simulink subsystem "Sub_Plant_And_Environments"  (R2020a)
settings: Solver=VariableStepAuto  StartTime=0.0  StopTime=10.0  RelTol=1e-3
values from neighbouring files (symbols this model uses):
  a_rad = deg2rad(a)    [plant_init.m]
  AF = [0.12, 0.22, 0.292]    [plant_init.m]
  l1 = [(D14(3)-RB(3)+PZ(1)*dz),     (D14(3)-RB(3)+PZ(1)*dz),     -hypot( D14(1)-RB(1), D14(2)-RB(2))]    [plant_init.m]
  l2 = [-(D14(3)-RB(3)+PZ(2)*dz),      (D14(3)-RB(3)+PZ(2)*dz),      -hypot( D14(1)+RB(1), D14(2)-RB(2))]    [plant_init.m]
  l3 = [(D14(3)-RB(3)+PZ(3)*dz),      (D14(3)-RB(3)+PZ(3)*dz),      hypot(D14(1)+RB(1), D14(2)+RB(2))]    [plant_init.m]
  l4 = [-(D14(3)-RB(3)+PZ(4)*dz),      (D14(3)-RB(3)+PZ(4)*dz),      hypot(D14(1)-RB(1), D14(2)+RB(2))]    [plant_init.m]
  l5 = [(D58(2)-RB(2)+PZ(1)*dz),      -(D58(1)-RB(1)+PZ(1)*dz), 0]    [plant_init.m]
  l6 = [-(D58(2)-RB(2)+PZ(2)*dz),       -(D58(1)+RB(1)+PZ(2)*dz), 0]    [plant_init.m]
  l7 = [-(D58(2)+RB(2)+PZ(3)*dz),     (D58(1)+RB(1)+PZ(3)*dz), 0]    [plant_init.m]
  l8 = [(D58(2)+RB(2)+PZ(4)*dz),      (D58(1)-RB(1)+PZ(2)*dz), 0]    [plant_init.m]
  mass = 33.95    [plant_init.m]
  N = T200Spec16V{:,6}    [InitController.m]    (also in plant_init.m)
  PWM = T200Spec16V{:,1}    [InitController.m]    (also in plant_init.m)
  RB = [ 0.001,      -0.003,       0.027]    [plant_init.m]
  RG = [ 0.001,      -0.003,       0.027]    [plant_init.m]
  rho = 998    [plant_init.m]
  volume = 0.027    [plant_init.m]
libraries: sharedtransform x11, vrlib x9, shared6dof x1, aerolibasang x1
(part 1 of 2)
settings Model: Creator=Lamarre  LastModifiedBy=Lamarre

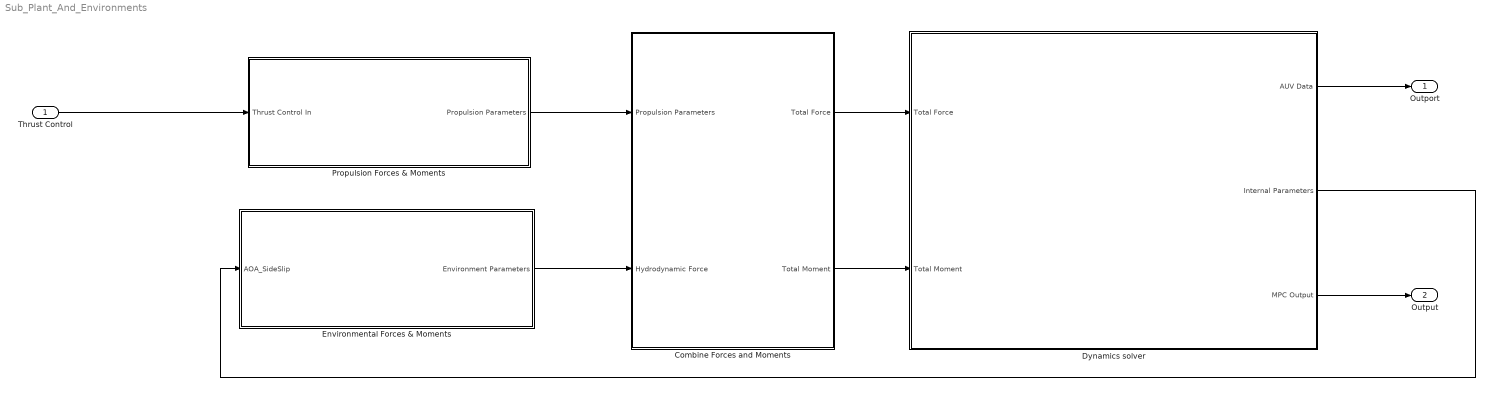
== system Sub_Plant_And_Environments ==
  Thrust Control : Inport
  Combine Forces and Moments : Subsystem
  Dynamics solver : Subsystem
  Environmental Forces & Moments : Subsystem
  Propulsion Forces & Moments : Subsystem
  Outport : Outport  VectorParamsAs1DForOutWhenUnconnected=off
  Output : Outport  Port=2
  wires:
  Dynamics solver/1(AUV Data) -> Outport/1
  Environmental Forces & Moments/1(Environment Parameters) -> Combine Forces and Moments/2(Hydrodynamic Force)
  Dynamics solver/2(Internal Parameters) -> Environmental Forces & Moments/1(AOA_SideSlip)
  Combine Forces and Moments/1(Total Force) -> Dynamics solver/1(Total Force)
  Thrust Control/1 -> Propulsion Forces & Moments/1(Thrust Control In)
  Propulsion Forces & Moments/1(Propulsion Parameters) -> Combine Forces and Moments/1(Propulsion Parameters)
  Dynamics solver/3(MPC Output) -> Output/1
  Combine Forces and Moments/2(Total Moment) -> Dynamics solver/2(Total Moment)

== system Sub_Plant_And_Environments/Combine Forces and Moments ==
  Propulsion Parameters : Inport
  Hydrodynamic Force : Inport  Port=2
  Bus Selector : BusSelector  OutputSignals=PropForce,PropMoment
  Bus Selector1 : BusSelector  OutputSignals=LDForce,HSForce,HS Moment
  Saturation : Saturate  UpperLimit=600  LowerLimit=-600
  Saturation1 : Saturate  UpperLimit=600  LowerLimit=-600
  Sum : Sum  Inputs=+++
  Sum1 : Sum  Inputs=|++
  Total Force : Outport  VectorParamsAs1DForOutWhenUnconnected=off
  Total Moment : Outport  Port=2  VectorParamsAs1DForOutWhenUnconnected=off
  wires:
  Bus Selector1/3 -> Sum1/2  "<HS Moment>"
  Bus Selector/2 -> Sum1/1  "<PropMoment>"
  Sum/1 -> Saturation/1
  Sum1/1 -> Total Moment/1
  Saturation1/1 -> Sum/2
  Saturation/1 -> Total Force/1
  Propulsion Parameters/1 -> Bus Selector/1
  Hydrodynamic Force/1 -> Bus Selector1/1
  Bus Selector/1 -> Sum/1  "<PropForce>"
  Bus Selector1/1 -> Saturation1/1  "<LDForce>"
  Bus Selector1/2 -> Sum/3  "<HSForce>"

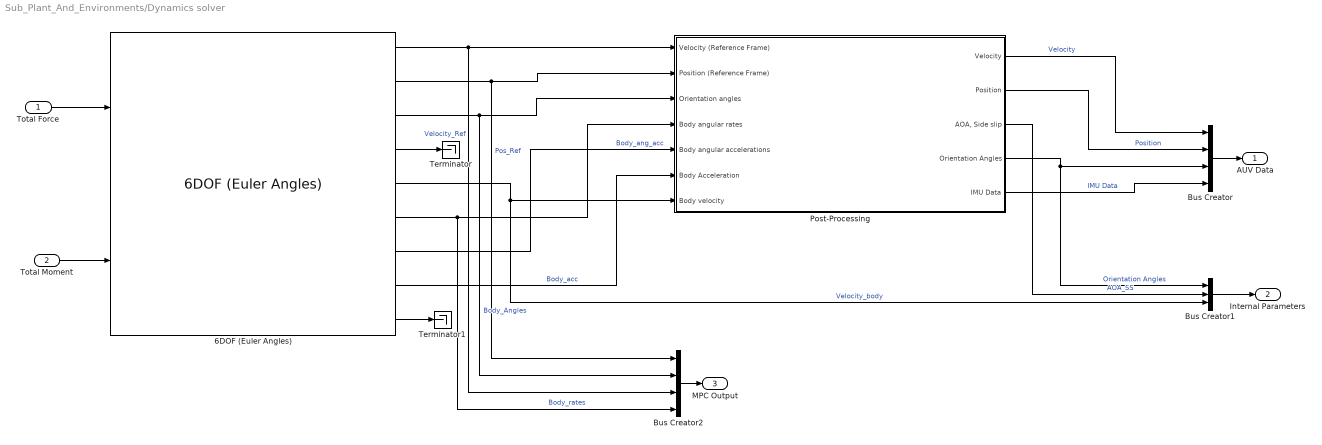
== system Sub_Plant_And_Environments/Dynamics solver ==
  Total Force : Inport
  Total Moment : Inport  Port=2
  6DOF (Euler Angles) : shared6dof/6DOF (Euler Angles)  units=Metric (MKS)  mtype=Fixed  rep=Euler Angles  xme_0=IP  Vm_0=IV  eul_0=IE  pm_0=IB  mass_0=mass  mass_e=0.5  mass_f=2.0  inertia=I  inertia_e=eye(3)  inertia_f=2*eye(3)  k_quat=1.0  vre_flag=on  abi_flag=on  aMode=0  xme_statename=''  Vm_statename=''  eul_statename=''  quat_statename=''  pm_statename=''  mass_statename=''
      settings: SourceProductBaseCode=AE,PW,MT,VE,VP
  Bus Creator : BusCreator  Inputs=4
  Bus Creator1 : BusCreator  Inputs=3
  Bus Creator2 : BusCreator  Inputs=4
  Post-Processing : Subsystem
  Terminator : Terminator
  Terminator1 : Terminator
  AUV Data : Outport  VectorParamsAs1DForOutWhenUnconnected=off
  Internal Parameters : Outport  Port=2  VectorParamsAs1DForOutWhenUnconnected=off
  MPC Output : Outport  Port=3
  wires:
  6DOF (Euler Angles)/6 -> Bus Creator2/4, Post-Processing/4(Body angular rates)  "Body_rates"
  Post-Processing/3("AOA, Side slip") -> Bus Creator1/2  "AOA_SS"
  6DOF (Euler Angles)/8 -> Post-Processing/6(Body Acceleration)  "Body_acc"
  Post-Processing/2(" Position") -> Bus Creator/2  "Position"
  6DOF (Euler Angles)/7 -> Post-Processing/5(Body angular accelerations)  "Body_ang_acc"
  6DOF (Euler Angles)/2 -> Bus Creator2/1, Post-Processing/2(Position (Reference Frame))  "Pos_Ref"
  6DOF (Euler Angles)/3 -> Bus Creator2/2, Post-Processing/3(Orientation angles)  "Body_Angles"
  Post-Processing/1(Velocity) -> Bus Creator/1  "Velocity"
  6DOF (Euler Angles)/1 -> Post-Processing/1(Velocity (Reference Frame)), Bus Creator2/3  "Velocity_Ref"
  6DOF (Euler Angles)/5 -> Bus Creator1/3, Post-Processing/7(Body velocity)  "Velocity_body"
  Post-Processing/4(Orientation Angles) -> Bus Creator1/1, Bus Creator/3  "Orientation Angles"
  Total Force/1 -> 6DOF (Euler Angles)/1
  Total Moment/1 -> 6DOF (Euler Angles)/2
  Bus Creator/1 -> AUV Data/1
  Bus Creator1/1 -> Internal Parameters/1
  6DOF (Euler Angles)/4 -> Terminator/1
  6DOF (Euler Angles)/9 -> Terminator1/1
  Post-Processing/5(IMU Data) -> Bus Creator/4  "IMU Data"
  Bus Creator2/1 -> MPC Output/1

== system Sub_Plant_And_Environments/Environmental Forces & Moments ==
  AOA_SideSlip : Inport
  Bus Creator : BusCreator  Inputs=3
  Bus Selector : BusSelector  OutputSignals=Velocity_body,AOA_SS,Orientation Angles
  Hydrodynamic Forces : Subsystem  Variant=on
  Hydrostatic Forces : Subsystem
  Environment Parameters : Outport  VectorParamsAs1DForOutWhenUnconnected=off
  wires:
  Hydrodynamic Forces/1("Force due to Lift, Drag") -> Bus Creator/1  "LDForce"
  Hydrostatic Forces/1(Hydrostatic Force) -> Bus Creator/2  "HSForce"
  Hydrostatic Forces/2(Hydrostatic Moment) -> Bus Creator/3  "HS Moment"
  Bus Creator/1 -> Environment Parameters/1
  AOA_SideSlip/1 -> Bus Selector/1
  Bus Selector/1 -> Hydrodynamic Forces/1("Submarine Velocity (Body Axis) ")  "<Velocity_body>"
  Bus Selector/2 -> Hydrodynamic Forces/2("AOA, Side Slip")  "<AOA_SS>"
  Bus Selector/3 -> Hydrostatic Forces/1(In1)  "<Orientation Angles>"

== system Sub_Plant_And_Environments/Propulsion Forces & Moments ==
  Thrust Control In : Inport
  Bus Creator : BusCreator  Inputs=2
  Force and moments due to Thrust : Subsystem
  Input commands to Thrust : Subsystem
  Propulsion Parameters : Outport  VectorParamsAs1DForOutWhenUnconnected=off
  wires:
  Input commands to Thrust/1(Thrust values) -> Force and moments due to Thrust/1(Thrust Inputs)
  Thrust Control In/1 -> Input commands to Thrust/1(Thrust Control Inputs)
  Force and moments due to Thrust/1(Propulsion Force) -> Bus Creator/1  "PropForce"
  Force and moments due to Thrust/2(Propulsion Moment) -> Bus Creator/2  "PropMoment"
  Bus Creator/1 -> Propulsion Parameters/1

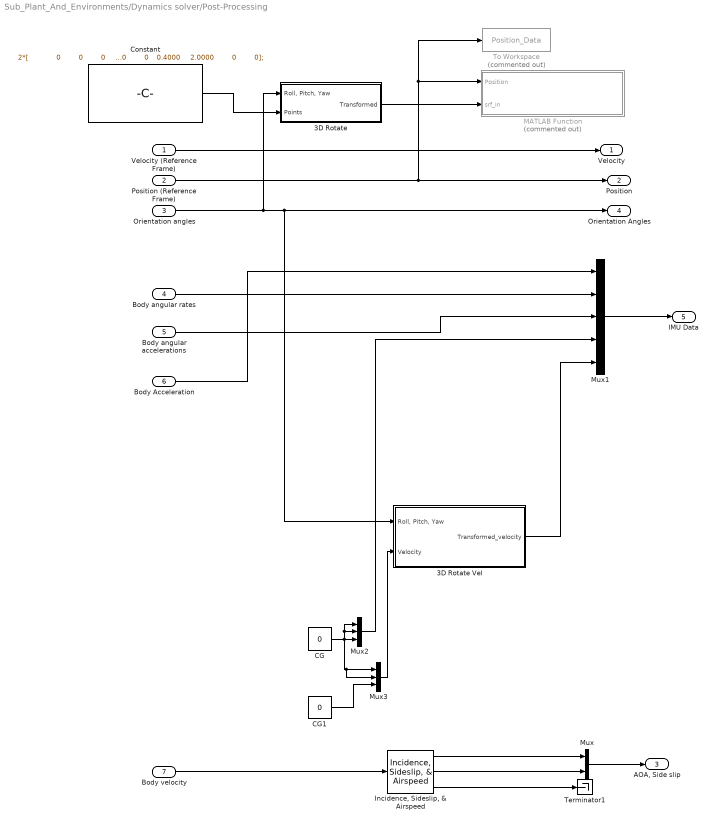
== system Sub_Plant_And_Environments/Dynamics solver/Post-Processing ==
  Velocity (Reference Frame) : Inport
  Position (Reference Frame) : Inport  Port=2
  Orientation angles : Inport  Port=3
  Body angular rates : Inport  Port=4
  Body angular accelerations : Inport  Port=5
  Body Acceleration : Inport  Port=6
  Body velocity : Inport  Port=7
  "3D Rotate " : Subsystem
  3D Rotate Vel : Subsystem
  CG : Constant  Value=0
  CG1 : Constant  Value=0
  Constant : Constant  Value=|
      | 2*[              0         0         0
      |     2.0000         0         0
      |     2.0000    0.4000         0
      |          0    0.4000         0
      |          0         0         0
      |          0         0    0.4000
      |     2.0000         0    0.4000
      |     2.0000    0.4000    0.4000
      |          0    0.4000    0.4000
      |          0         0    0.4000
      |          0    0.4000    0.4000
      |          0    0.4000         0
      |     2.0000    0.4000         0
      |     2.0000    0.4000    0.4000
      |     2.0000         0    0.4000
      |     2.0000         0         0];
  "Incidence, Sideslip, & Airspeed" : aerolibasang/Incidence, Sideslip, & Airspeed
  MATLAB Function : MATLAB Function  Commented=on  TreatAsAtomicUnit=on  SystemSampleTime=0.05
  Mux : Mux  Inputs=2
  Mux1 : Mux  Inputs=5
  Mux2 : Mux  Inputs=3
  Mux3 : Mux  Inputs=3
  Terminator1 : Terminator
  To Workspace : ToWorkspace  Commented=on  VariableName=Position_Data  SampleTime=-1
  Velocity : Outport  VectorParamsAs1DForOutWhenUnconnected=off
  " Position" : Outport  Port=2  VectorParamsAs1DForOutWhenUnconnected=off
  "AOA, Side slip" : Outport  Port=3  VectorParamsAs1DForOutWhenUnconnected=off
  Orientation Angles : Outport  Port=4  VectorParamsAs1DForOutWhenUnconnected=off
  IMU Data : Outport  Port=5  VectorParamsAs1DForOutWhenUnconnected=off
  wires:
  Body angular accelerations/1 -> Mux1/3
  "Incidence, Sideslip, & Airspeed"/2 -> Mux/2
  Body velocity/1 -> "Incidence, Sideslip, & Airspeed"/1
  "Incidence, Sideslip, & Airspeed"/1 -> Mux/1
  Body angular rates/1 -> Mux1/2
  CG/1 -> Mux3/2, Mux3/1, Mux2/3, Mux2/2, Mux2/1
  3D Rotate Vel/1("Transformed_velocity ") -> Mux1/5
  Mux2/1 -> Mux1/4
  Position (Reference Frame)/1 -> To Workspace/1, MATLAB Function/1(Position), " Position"/1
  Mux/1 -> "AOA, Side slip"/1
  CG1/1 -> Mux3/3
  Mux3/1 -> 3D Rotate Vel/2(Velocity)
  Body Acceleration/1 -> Mux1/1
  Velocity (Reference Frame)/1 -> Velocity/1
  Orientation angles/1 -> 3D Rotate Vel/1("Roll, Pitch, Yaw"), Orientation Angles/1, "3D Rotate "/1("Roll, Pitch, Yaw")
  Mux1/1 -> IMU Data/1
  Constant/1 -> "3D Rotate "/2(Points)
  "3D Rotate "/1("Transformed ") -> MATLAB Function/2(srf_in)
  "Incidence, Sideslip, & Airspeed"/3 -> Terminator1/1

== system Sub_Plant_And_Environments/Environmental Forces & Moments/Hydrodynamic Forces ==
  "Submarine Velocity (Body Axis) " : Inport
  "AOA, Side Slip" : Inport  Port=2
  Hydrodynamic Forces - Accurate : Subsystem  VariantControl=c==1
  Hydrodynamic Forces - Basic : Subsystem  VariantControl=c==0
  "Force due to Lift, Drag" : Outport  VectorParamsAs1DForOutWhenUnconnected=off

== system Sub_Plant_And_Environments/Environmental Forces & Moments/Hydrostatic Forces ==
  In1 : Inport
  Constant : Constant
  Environment Model : Subsystem  mask{ro=rho, V=volume, M=mass, a=RG(1)-RB(1), b=RG(2)-RB(2), c=RG(3)-RB(3)}
      mask prompts: ro "Density of Water"; V "Volume of Submarine"; M "Mass of Submarine"; a "X Distance between CG and CB"; b "Y Distance between CG and CB"; c "Z Distance between CG and CB"
      mask DialogControl DescTextVar Prompt: Enter the Submarine related Parameters
      mask DialogControl Container3 Prompt: Distance between CG and Center of Buoyancy
  Hydrostatic Force : Outport  VectorParamsAs1DForOutWhenUnconnected=off
  Hydrostatic Moment : Outport  Port=2  VectorParamsAs1DForOutWhenUnconnected=off
  wires:
  Constant/1 -> Environment Model/1("Fraction submerged ")
  Environment Model/2(Moment due to Weight and Buoyancy) -> Hydrostatic Moment/1
  Environment Model/1(Forces due to Weight and Buoyancy) -> Hydrostatic Force/1
  In1/1 -> Environment Model/2(Orientation Angles)

== system Sub_Plant_And_Environments/Propulsion Forces & Moments/Force and moments due to Thrust ==
  Thrust Inputs : Inport
  "Thrust to Propulsion " : Subsystem
  Propulsion Force : Outport  VectorParamsAs1DForOutWhenUnconnected=off
  Propulsion Moment : Outport  Port=2  VectorParamsAs1DForOutWhenUnconnected=off
  wires:
  "Thrust to Propulsion "/2(Propulsion Moment) -> Propulsion Moment/1
  Thrust Inputs/1 -> "Thrust to Propulsion "/1(Thrust Inputs)
  "Thrust to Propulsion "/1(Propulsion Force) -> Propulsion Force/1

== system Sub_Plant_And_Environments/Propulsion Forces & Moments/Input commands to Thrust ==
  Thrust Control Inputs : Inport
  Demux : Demux  Outputs=8
  "PWM Signals to Thrust " : Subsystem
  Subsystem : Subsystem
  Thrust values : Outport  VectorParamsAs1DForOutWhenUnconnected=off
  wires:
  Subsystem/2(Moteur 2) -> "PWM Signals to Thrust "/2(PWM Moteur 2)
  Subsystem/1(Moteur 1) -> "PWM Signals to Thrust "/1(PWM Moteur 1)
  "PWM Signals to Thrust "/1(Thrust (N)) -> Thrust values/1
  Thrust Control Inputs/1 -> Demux/1
  Subsystem/8(Moteur 8) -> "PWM Signals to Thrust "/8("PWM Moteur 8 ")
  Subsystem/7(Moteur 7) -> "PWM Signals to Thrust "/7(PWM Moteur 7)
  Subsystem/6(Moteur 6) -> "PWM Signals to Thrust "/6(PWM Moteur 6)
  Subsystem/5(Moteur 5) -> "PWM Signals to Thrust "/5("PWM Moteur 5 ")
  Subsystem/4(Moteur 4) -> "PWM Signals to Thrust "/4(PWM Moteur 4)
  Subsystem/3(Moteur 3) -> "PWM Signals to Thrust "/3(PWM Moteur 3)
  Demux/1 -> Subsystem/1(Force M1)  "Force Moteur 1"
  Demux/2 -> Subsystem/2(Force M2)  "Force Moteur 2"
  Demux/3 -> Subsystem/3(Force M3)  "Force Moteur 3"
  Demux/4 -> Subsystem/4(Force M4)  "Force Moteur 4"
  Demux/5 -> Subsystem/5(Force M5)  "Force Moteur 5"
  Demux/6 -> Subsystem/6(Force M6)  "Force Moteur 6"
  Demux/7 -> Subsystem/7(Force M7)  "Force Moteur 7"
  Demux/8 -> Subsystem/8(Force M8)  "Force Moteur 8"

== system Sub_Plant_And_Environments/Dynamics solver/Post-Processing/3D Rotate  ==
  "Roll, Pitch, Yaw" : Inport
  Points : Inport  Port=2
  Gain : Gain
  Matrix Multiply : Product  Multiplication=Matrix(*)
  Rotation Angles to Direction Cosine Matrix : sharedtransform/Rotation Angles to Direction Cosine Matrix  rotationOrder=XYZ  aMode=aMode
      settings: SourceProductBaseCode=AE,PW,MT,VE,VP
  Transpose : Math  Operator=transpose  SignedPower=on  SaturateOnIntegerOverflow=on
  "Transformed " : Outport  VectorParamsAs1DForOutWhenUnconnected=off
  wires:
  Matrix Multiply/1 -> "Transformed "/1
  Rotation Angles to Direction Cosine Matrix/1 -> Transpose/1
  Points/1 -> Matrix Multiply/1
  "Roll, Pitch, Yaw"/1 -> Gain/1
  Transpose/1 -> Matrix Multiply/2
  Gain/1 -> Rotation Angles to Direction Cosine Matrix/1

== system Sub_Plant_And_Environments/Dynamics solver/Post-Processing/3D Rotate Vel ==
  "Roll, Pitch, Yaw" : Inport
  Velocity : Inport  Port=2
  Gain : Gain
  Matrix Multiply : Product  Multiplication=Matrix(*)
  Rotation Angles to Direction Cosine Matrix : sharedtransform/Rotation Angles to Direction Cosine Matrix  rotationOrder=XYZ  aMode=aMode
      settings: SourceProductBaseCode=AE,PW,MT,VE,VP
  Transpose : Math  Operator=transpose  SignedPower=on  SaturateOnIntegerOverflow=on
  "Transformed_velocity " : Outport  VectorParamsAs1DForOutWhenUnconnected=off
  wires:
  Matrix Multiply/1 -> "Transformed_velocity "/1
  Rotation Angles to Direction Cosine Matrix/1 -> Transpose/1
  Velocity/1 -> Matrix Multiply/2
  "Roll, Pitch, Yaw"/1 -> Gain/1
  Transpose/1 -> Matrix Multiply/1
  Gain/1 -> Rotation Angles to Direction Cosine Matrix/1

== system Sub_Plant_And_Environments/Environmental Forces & Moments/Hydrodynamic Forces/Hydrodynamic Forces - Accurate ==
  note: Source of Equations:
      | Submarine Dynamic Modeling, by
      | Dr Peter Ridley Julien Fontan and Dr Peter Corke
      |
      | Part: Hydrodynamic forces and moments
  "Submarine Velocity (Body Axis) " : Inport
  "AOA, Side Slip" : Inport  Port=2
  Force Exerted due to Drag (Body Axis) : Subsystem
  Force Exerted due to Lift (Body Axis) : Subsystem
  Sum : Sum
  "Force due to Lift, Drag" : Outport  VectorParamsAs1DForOutWhenUnconnected=off
  wires:
  Force Exerted due to Drag (Body Axis)/1(Drag Forces in Body Axis) -> Sum/1
  Force Exerted due to Lift (Body Axis)/1(Lift Forces in Body Axis) -> Sum/2
  "AOA, Side Slip"/1 -> Force Exerted due to Drag (Body Axis)/2(AOA and Side Slip), Force Exerted due to Lift (Body Axis)/2(AOA and Side Slip)
  "Submarine Velocity (Body Axis) "/1 -> Force Exerted due to Lift (Body Axis)/1(Marine Velocities in Body Axis), Force Exerted due to Drag (Body Axis)/1(Marine Velocities in Body Axis)
  Sum/1 -> "Force due to Lift, Drag"/1

== system Sub_Plant_And_Environments/Environmental Forces & Moments/Hydrodynamic Forces/Hydrodynamic Forces - Basic ==
  "Submarine Velocity (Body Axis) " : Inport
  "AOA, Side Slip" : Inport  Port=2
  Force Exerted due to Drag (Body Axis) : Subsystem
  Force Exerted due to Lift (Body Axis) : Subsystem
  Sum : Sum
  "Force due to Lift, Drag" : Outport  VectorParamsAs1DForOutWhenUnconnected=off
  wires:
  Force Exerted due to Drag (Body Axis)/1(Drag Forces in Body Axis) -> Sum/1
  Force Exerted due to Lift (Body Axis)/1(Lift Forces in Body Axis) -> Sum/2
  "AOA, Side Slip"/1 -> Force Exerted due to Drag (Body Axis)/2(AOA and Side Slip), Force Exerted due to Lift (Body Axis)/2(AOA and Side Slip)
  "Submarine Velocity (Body Axis) "/1 -> Force Exerted due to Lift (Body Axis)/1(Marine Velocities in Body Axis), Force Exerted due to Drag (Body Axis)/1(Marine Velocities in Body Axis)
  Sum/1 -> "Force due to Lift, Drag"/1

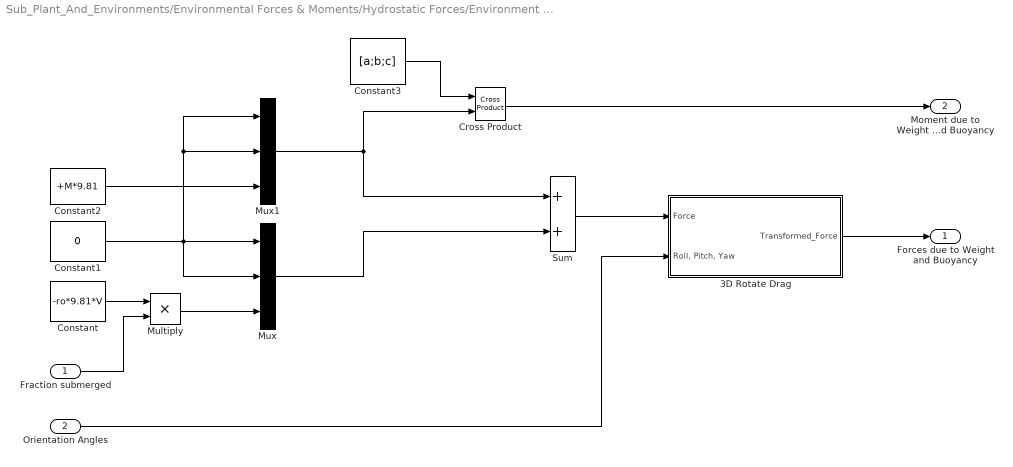
== system Sub_Plant_And_Environments/Environmental Forces & Moments/Hydrostatic Forces/Environment Model ==
  "Fraction submerged " : Inport
  Orientation Angles : Inport  Port=2
  3D Rotate Drag : Subsystem
  Constant : Constant  Value=-ro*9.81*V
  Constant1 : Constant  Value=0
  Constant2 : Constant  Value=+M*9.81
  Constant3 : Constant  Value=[a;b;c]
  Cross Product : vrlib/Utilities/Cross Product
  Multiply : Product
  Mux : Mux  Inputs=3
  Mux1 : Mux  Inputs=3
  Sum : Sum
  Forces due to Weight and Buoyancy : Outport  VectorParamsAs1DForOutWhenUnconnected=off
  Moment due to Weight and Buoyancy : Outport  Port=2  VectorParamsAs1DForOutWhenUnconnected=off
  wires:
  Cross Product/1 -> Moment due to Weight and Buoyancy/1
  Constant3/1 -> Cross Product/1
  "Fraction submerged "/1 -> Multiply/2
  Mux/1 -> Sum/2
  Multiply/1 -> Mux/3
  Mux1/1 -> Sum/1, Cross Product/2
  Constant/1 -> Multiply/1
  Constant1/1 -> Mux/1, Mux/2, Mux1/2, Mux1/1
  Constant2/1 -> Mux1/3
  Sum/1 -> 3D Rotate Drag/1(Force)
  Orientation Angles/1 -> 3D Rotate Drag/2("Roll, Pitch, Yaw")
  3D Rotate Drag/1("Transformed_Force ") -> Forces due to Weight and Buoyancy/1

== system Sub_Plant_And_Environments/Propulsion Forces & Moments/Force and moments due to Thrust/Thrust to Propulsion  ==
  Thrust Inputs : Inport
  Demux : Demux  Outputs=8
  Moment computation : Subsystem
  Sum : Sum  Inputs=++++++++
  Thrust Transformation : Subsystem
  Propulsion Force : Outport  VectorParamsAs1DForOutWhenUnconnected=off
  Propulsion Moment : Outport  Port=2  VectorParamsAs1DForOutWhenUnconnected=off
  wires:
  Demux/5 -> Moment computation/5(Moteur 5)
  Demux/4 -> Moment computation/4(Moteur 4)
  Demux/3 -> Moment computation/3(Moteur 3)
  Demux/2 -> Moment computation/2(Moteur 2)
  Demux/1 -> Moment computation/1(Moteur 1)
  Thrust Transformation/3(Thrust M3) -> Sum/3
  Moment computation/1(Moment) -> Propulsion Moment/1
  Thrust Transformation/4(Thrust M4) -> Sum/4
  Thrust Transformation/5(Thrust M5) -> Sum/5
  Sum/1 -> Propulsion Force/1
  Thrust Inputs/1 -> Thrust Transformation/1(Thrust Inputs), Demux/1
  Thrust Transformation/1(Thrust M1) -> Sum/1
  Thrust Transformation/2(Thrust M2) -> Sum/2
  Demux/6 -> Moment computation/6(Moteur 6)
  Demux/7 -> Moment computation/7(Moteur 7)
  Demux/8 -> Moment computation/8(Moteur 8)
  Thrust Transformation/6(Thrust M6) -> Sum/6
  Thrust Transformation/7(Thrust M7) -> Sum/7
  Thrust Transformation/8(Thrust M8) -> Sum/8

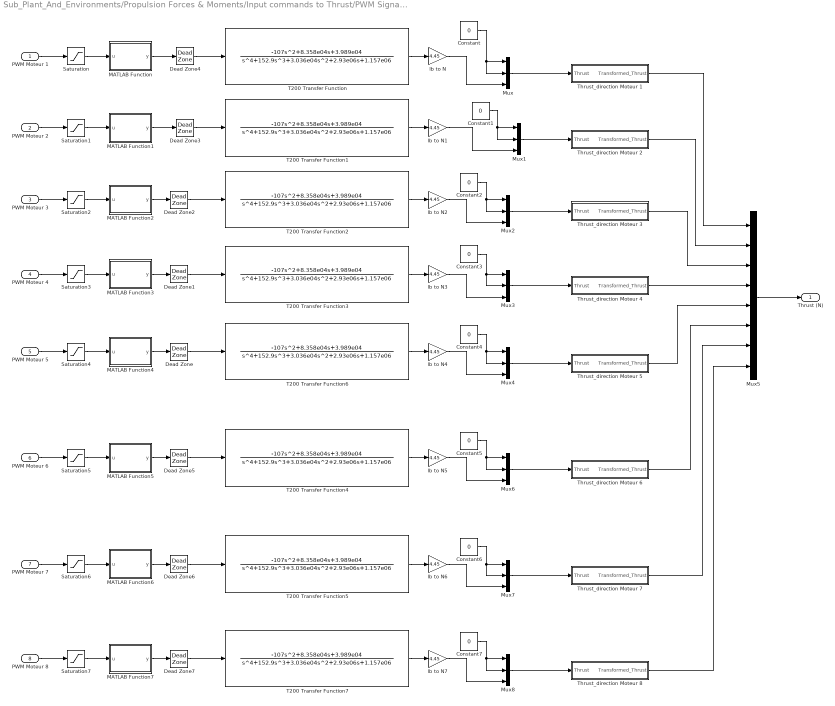
== system Sub_Plant_And_Environments/Propulsion Forces & Moments/Input commands to Thrust/PWM Signals to Thrust  ==
  PWM Moteur 1 : Inport
  PWM Moteur 2 : Inport  Port=2
  PWM Moteur 3 : Inport  Port=3
  PWM Moteur 4 : Inport  Port=4
  "PWM Moteur 5 " : Inport  Port=5
  PWM Moteur 6 : Inport  Port=6
  PWM Moteur 7 : Inport  Port=7
  "PWM Moteur 8 " : Inport  Port=8
  Constant{,1..7} (8 alike) : Constant  Value=0
  Dead Zone{,2..7} (7 alike) : DeadZone  LowerValue=-10  UpperValue=+10  SaturateOnIntegerOverflow=on
  Dead Zone1 : DeadZone  LowerValue=-10  UpperValue=10  SaturateOnIntegerOverflow=on
  MATLAB Function : MATLAB Function  TreatAsAtomicUnit=on
  MATLAB Function1 : MATLAB Function  TreatAsAtomicUnit=on
  MATLAB Function2 : MATLAB Function  TreatAsAtomicUnit=on
  MATLAB Function3 : MATLAB Function  TreatAsAtomicUnit=on
  MATLAB Function4 : MATLAB Function  TreatAsAtomicUnit=on
  MATLAB Function5 : MATLAB Function  TreatAsAtomicUnit=on
  MATLAB Function6 : MATLAB Function  TreatAsAtomicUnit=on
  MATLAB Function7 : MATLAB Function  TreatAsAtomicUnit=on
  Mux{,1..4,6..8} (8 alike) : Mux  Inputs=3
  Mux5 : Mux  Inputs=8
  Saturation{,1..7} (8 alike) : Saturate  UpperLimit=1900  LowerLimit=1100
  T200 Transfer Function{,1..7} (8 alike) : TransferFcn  Numerator="[-107  8.358e04  3.989e04]"  Denominator="[1 152.9  3.036e04  2.93e06  1.157e06]"
  Thrust_direction Moteur 1 : Subsystem
  Thrust_direction Moteur 2 : Subsystem
  Thrust_direction Moteur 3 : Subsystem
  Thrust_direction Moteur 4 : Subsystem
  Thrust_direction Moteur 5 : Subsystem
  Thrust_direction Moteur 6 : Subsystem
  Thrust_direction Moteur 7 : Subsystem
  Thrust_direction Moteur 8 : Subsystem
  lb to N{,1..7} (8 alike) : Gain  Gain=4.45
  Thrust (N) : Outport  VectorParamsAs1DForOutWhenUnconnected=off
  wires:
  Thrust_direction Moteur 1/1("Transformed_Thrust ") -> Mux5/1
  Thrust_direction Moteur 2/1("Transformed_Thrust ") -> Mux5/2
  Thrust_direction Moteur 8/1("Transformed_Thrust ") -> Mux5/8
  Thrust_direction Moteur 7/1("Transformed_Thrust ") -> Mux5/7
  Thrust_direction Moteur 6/1("Transformed_Thrust ") -> Mux5/6
  Dead Zone7/1 -> T200 Transfer Function7/1
  Constant7/1 -> Mux8/2, Mux8/1
  Saturation7/1 -> MATLAB Function7/1(u)
  Mux8/1 -> Thrust_direction Moteur 8/1(Thrust)
  lb to N7/1 -> Mux8/3
  MATLAB Function7/1(y) -> Dead Zone7/1
  T200 Transfer Function7/1 -> lb to N7/1
  "PWM Moteur 8 "/1 -> Saturation7/1
  Dead Zone6/1 -> T200 Transfer Function5/1
  Constant6/1 -> Mux7/2, Mux7/1
  Saturation6/1 -> MATLAB Function6/1(u)
  Mux7/1 -> Thrust_direction Moteur 7/1(Thrust)
  lb to N6/1 -> Mux7/3
  MATLAB Function6/1(y) -> Dead Zone6/1
  T200 Transfer Function5/1 -> lb to N6/1
  PWM Moteur 7/1 -> Saturation6/1
  Dead Zone5/1 -> T200 Transfer Function4/1
  Constant5/1 -> Mux6/2, Mux6/1
  Saturation5/1 -> MATLAB Function5/1(u)
  Mux6/1 -> Thrust_direction Moteur 6/1(Thrust)
  lb to N5/1 -> Mux6/3
  MATLAB Function5/1(y) -> Dead Zone5/1
  T200 Transfer Function4/1 -> lb to N5/1
  PWM Moteur 6/1 -> Saturation5/1
  Dead Zone4/1 -> T200 Transfer Function/1
  Dead Zone3/1 -> T200 Transfer Function1/1
  Dead Zone2/1 -> T200 Transfer Function2/1
  Dead Zone1/1 -> T200 Transfer Function3/1
  Dead Zone/1 -> T200 Transfer Function6/1
  MATLAB Function4/1(y) -> Dead Zone/1
  MATLAB Function3/1(y) -> Dead Zone1/1
  MATLAB Function2/1(y) -> Dead Zone2/1
  MATLAB Function1/1(y) -> Dead Zone3/1
  Saturation3/1 -> MATLAB Function3/1(u)
  PWM Moteur 4/1 -> Saturation3/1
  Saturation4/1 -> MATLAB Function4/1(u)
  Saturation2/1 -> MATLAB Function2/1(u)
  Saturation1/1 -> MATLAB Function1/1(u)
  Saturation/1 -> MATLAB Function/1(u)
  MATLAB Function/1(y) -> Dead Zone4/1
  T200 Transfer Function3/1 -> lb to N3/1
  lb to N2/1 -> Mux2/3
  Mux4/1 -> Thrust_direction Moteur 5/1(Thrust)
  Mux5/1 -> Thrust (N)/1
  Thrust_direction Moteur 5/1("Transformed_Thrust ") -> Mux5/5
  lb to N/1 -> Mux/3
  Constant1/1 -> Mux1/2, Mux1/1
  T200 Transfer Function1/1 -> lb to N1/1
  Mux3/1 -> Thrust_direction Moteur 4/1(Thrust)
  "PWM Moteur 5 "/1 -> Saturation4/1
  PWM Moteur 1/1 -> Saturation/1
  Constant/1 -> Mux/2, Mux/1
  Thrust_direction Moteur 4/1("Transformed_Thrust ") -> Mux5/4
  Thrust_direction Moteur 3/1("Transformed_Thrust ") -> Mux5/3
  PWM Moteur 3/1 -> Saturation2/1
  Mux1/1 -> Thrust_direction Moteur 2/1(Thrust)
  lb to N1/1 -> Mux1/3
  lb to N4/1 -> Mux4/3
  Constant4/1 -> Mux4/2, Mux4/1
  T200 Transfer Function6/1 -> lb to N4/1
  Mux/1 -> Thrust_direction Moteur 1/1(Thrust)
  T200 Transfer Function/1 -> lb to N/1
  Constant2/1 -> Mux2/2, Mux2/1
  Mux2/1 -> Thrust_direction Moteur 3/1(Thrust)
  PWM Moteur 2/1 -> Saturation1/1
  Constant3/1 -> Mux3/2, Mux3/1
  lb to N3/1 -> Mux3/3
  T200 Transfer Function2/1 -> lb to N2/1

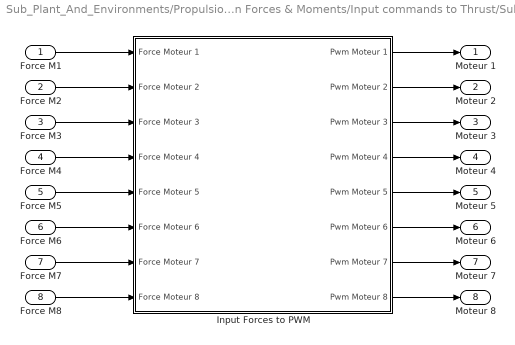
== system Sub_Plant_And_Environments/Propulsion Forces & Moments/Input commands to Thrust/Subsystem ==
  Force M1 : Inport
  Force M2 : Inport  Port=2
  Force M3 : Inport  Port=3
  Force M4 : Inport  Port=4
  Force M5 : Inport  Port=5
  Force M6 : Inport  Port=6
  Force M7 : Inport  Port=7
  Force M8 : Inport  Port=8
  Input Forces to PWM : Subsystem
  Moteur 1 : Outport
  Moteur 2 : Outport  Port=2
  Moteur 3 : Outport  Port=3
  Moteur 4 : Outport  Port=4
  Moteur 5 : Outport  Port=5
  Moteur 6 : Outport  Port=6
  Moteur 7 : Outport  Port=7
  Moteur 8 : Outport  Port=8
  wires:
  Input Forces to PWM/1(Pwm Moteur 1) -> Moteur 1/1
  Force M1/1 -> Input Forces to PWM/1(Force Moteur 1)
  Input Forces to PWM/2(Pwm Moteur 2) -> Moteur 2/1
  Input Forces to PWM/3(Pwm Moteur 3) -> Moteur 3/1
  Input Forces to PWM/4(Pwm Moteur 4) -> Moteur 4/1
  Input Forces to PWM/5(Pwm Moteur 5) -> Moteur 5/1
  Input Forces to PWM/6(Pwm Moteur 6) -> Moteur 6/1
  Input Forces to PWM/7(Pwm Moteur 7) -> Moteur 7/1
  Input Forces to PWM/8(Pwm Moteur 8) -> Moteur 8/1
  Force M2/1 -> Input Forces to PWM/2(Force Moteur 2)
  Force M3/1 -> Input Forces to PWM/3(Force Moteur 3)
  Force M4/1 -> Input Forces to PWM/4(Force Moteur 4)
  Force M5/1 -> Input Forces to PWM/5(Force Moteur 5)
  Force M6/1 -> Input Forces to PWM/6(Force Moteur 6)
  Force M7/1 -> Input Forces to PWM/7(Force Moteur 7)
  Force M8/1 -> Input Forces to PWM/8(Force Moteur 8)

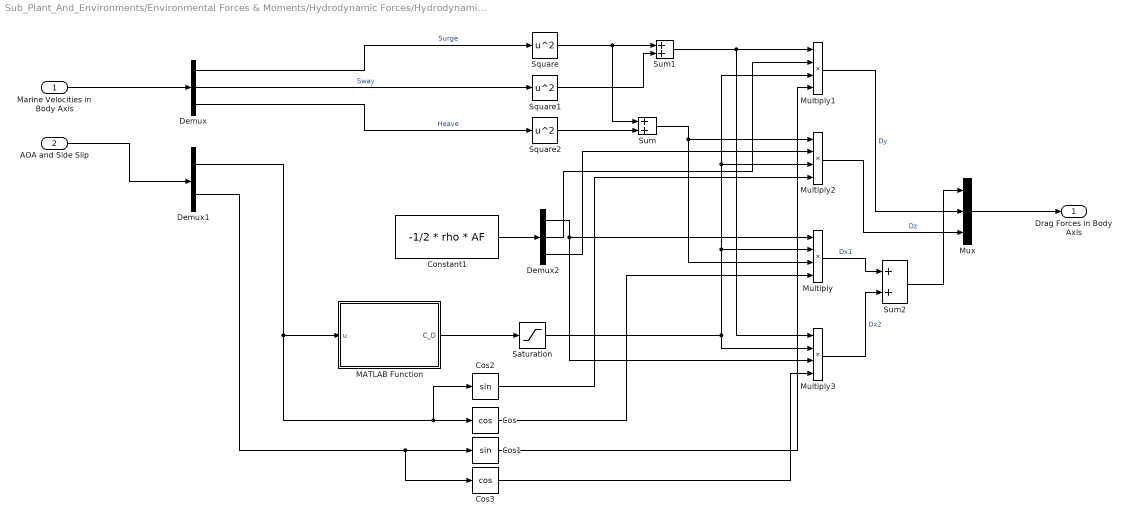
== system Sub_Plant_And_Environments/Environmental Forces & Moments/Hydrodynamic Forces/Hydrodynamic Forces - Accurate/Force Exerted due to Drag (Body Axis) ==
  Marine Velocities in Body Axis : Inport
  AOA and Side Slip : Inport  Port=2
  Constant1 : Constant  Value=-1/2 * rho * AF
  Cos : Trigonometry  Operator=cos
  Cos1 : Trigonometry
  Cos2 : Trigonometry
  Cos3 : Trigonometry  Operator=cos
  Demux : Demux  Outputs=3
  Demux1 : Demux  Outputs=2
  Demux2 : Demux  Outputs=3
  MATLAB Function : MATLAB Function  TreatAsAtomicUnit=on
  Multiply{,1..3} (4 alike) : Product  Inputs=4
  Mux : Mux  Inputs=3
  Saturation : Saturate  UpperLimit=25  LowerLimit=-25
  Square : Math  Operator=square  SignedPower=on  SaturateOnIntegerOverflow=on
  Square1 : Math  Operator=square  SignedPower=on  SaturateOnIntegerOverflow=on
  Square2 : Math  Operator=square  SignedPower=on  SaturateOnIntegerOverflow=on
  Sum : Sum
  Sum1 : Sum
  Sum2 : Sum
  Drag Forces in Body Axis : Outport  VectorParamsAs1DForOutWhenUnconnected=off
  wires:
  Saturation/1 -> Multiply/2, Multiply2/3, Multiply1/3, Multiply3/2
  Square1/1 -> Sum1/2
  Multiply1/1 -> Mux/2  "Dy"
  Sum2/1 -> Mux/1
  Cos3/1 -> Multiply3/4
  AOA and Side Slip/1 -> Demux1/1
  Marine Velocities in Body Axis/1 -> Demux/1
  Cos2/1 -> Multiply2/4
  Mux/1 -> Drag Forces in Body Axis/1
  Square2/1 -> Sum/2
  Demux1/2 -> Cos1/1, Cos3/1
  Demux1/1 -> MATLAB Function/1(u), Cos2/1, Cos/1
  MATLAB Function/1(C_D) -> Saturation/1
  Multiply2/1 -> Mux/3  "Dz"
  Cos/1 -> Multiply/4
  Demux/3 -> Square2/1  "Heave"
  Multiply3/1 -> Sum2/2  "Dx2"
  Sum/1 -> Multiply/3, Multiply2/1
  Demux/1 -> Square/1  "Surge"
  Multiply/1 -> Sum2/1  "Dx1"
  Sum1/1 -> Multiply1/1, Multiply3/1
  Cos1/1 -> Multiply1/4
  Demux/2 -> Square1/1  "Sway"
  Square/1 -> Sum1/1, Sum/1
  Constant1/1 -> Demux2/1
  Demux2/1 -> Multiply/1, Multiply3/3
  Demux2/2 -> Multiply1/2
  Demux2/3 -> Multiply2/2

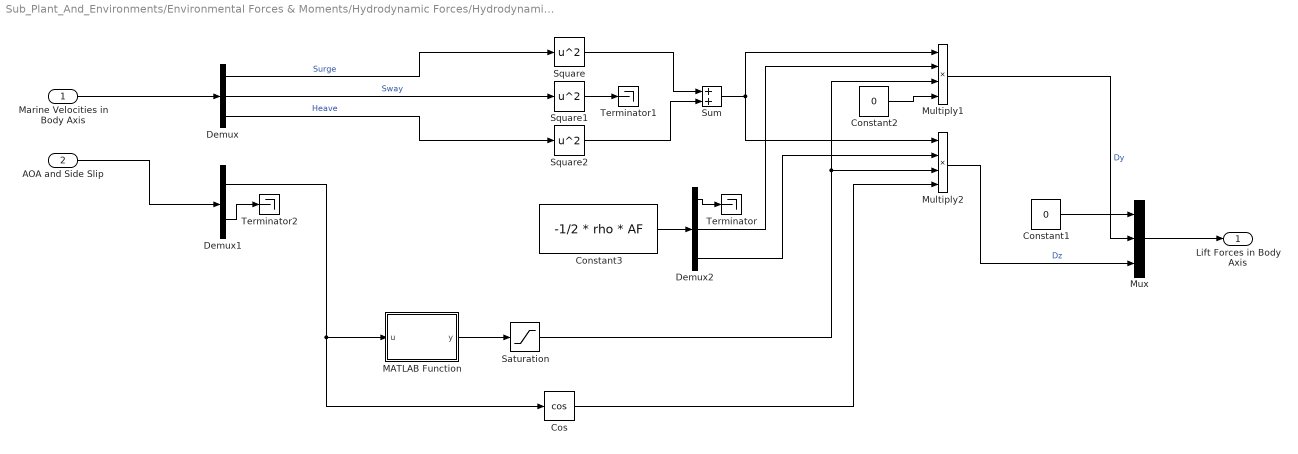
== system Sub_Plant_And_Environments/Environmental Forces & Moments/Hydrodynamic Forces/Hydrodynamic Forces - Accurate/Force Exerted due to Lift (Body Axis) ==
  Marine Velocities in Body Axis : Inport
  AOA and Side Slip : Inport  Port=2
  Constant1 : Constant  Value=0
  Constant2 : Constant  Value=0
  Constant3 : Constant  Value=-1/2 * rho * AF
  Cos : Trigonometry  Operator=cos
  Demux : Demux  Outputs=3
  Demux1 : Demux  Outputs=2
  Demux2 : Demux  Outputs=3
  MATLAB Function : MATLAB Function  TreatAsAtomicUnit=on
  Multiply1 : Product  Inputs=4
  Multiply2 : Product  Inputs=4
  Mux : Mux  Inputs=3
  Saturation : Saturate  UpperLimit=25  LowerLimit=-25
  Square : Math  Operator=square  SignedPower=on  SaturateOnIntegerOverflow=on
  Square1 : Math  Operator=square  SignedPower=on  SaturateOnIntegerOverflow=on
  Square2 : Math  Operator=square  SignedPower=on  SaturateOnIntegerOverflow=on
  Sum : Sum
  Terminator : Terminator
  Terminator1 : Terminator
  Terminator2 : Terminator
  Lift Forces in Body Axis : Outport  VectorParamsAs1DForOutWhenUnconnected=off
  wires:
  Saturation/1 -> Multiply2/3, Multiply1/3
  Constant2/1 -> Multiply1/4
  Multiply2/1 -> Mux/3  "Dz"
  Constant1/1 -> Mux/1
  Cos/1 -> Multiply2/4
  Square/1 -> Sum/1
  Demux/2 -> Square1/1  "Sway"
  Demux/1 -> Square/1  "Surge"
  Sum/1 -> Multiply1/1, Multiply2/1
  Multiply1/1 -> Mux/2  "Dy"
  Demux/3 -> Square2/1  "Heave"
  MATLAB Function/1(y) -> Saturation/1
  Demux1/1 -> MATLAB Function/1(u), Cos/1
  Square2/1 -> Sum/2
  Mux/1 -> Lift Forces in Body Axis/1
  Marine Velocities in Body Axis/1 -> Demux/1
  AOA and Side Slip/1 -> Demux1/1
  Square1/1 -> Terminator1/1
  Demux1/2 -> Terminator2/1
  Constant3/1 -> Demux2/1
  Demux2/2 -> Multiply1/2
  Demux2/3 -> Multiply2/2
  Demux2/1 -> Terminator/1

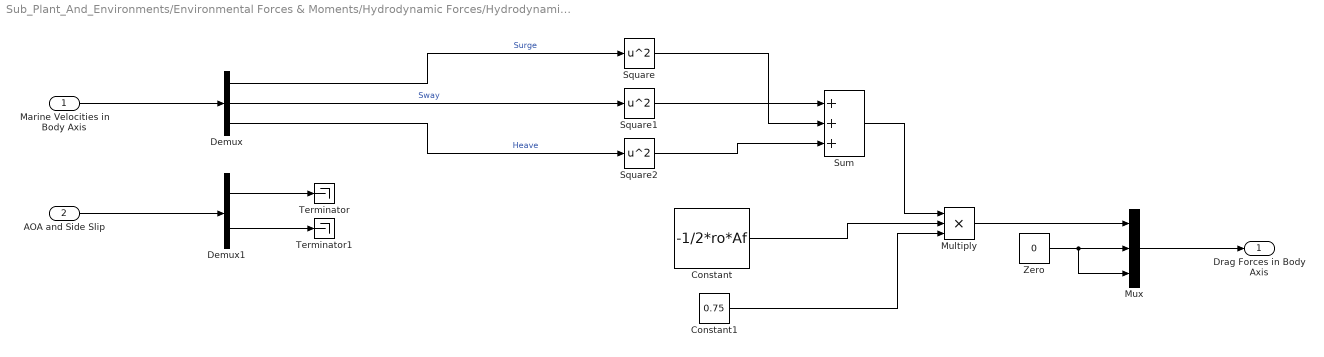
== system Sub_Plant_And_Environments/Environmental Forces & Moments/Hydrodynamic Forces/Hydrodynamic Forces - Basic/Force Exerted due to Drag (Body Axis) ==
  Marine Velocities in Body Axis : Inport
  AOA and Side Slip : Inport  Port=2
  Constant : Constant  Value=-1/2*ro*Af  mask{ro=rho, Af=AF(1)}
      mask prompts: ro "Density of Water"; Af "Submarine Frontal Area"
      mask DialogControl DescGroupVar Prompt: Input
      mask DialogControl DescTextVar Prompt: Enter the following values :
  Constant1 : Constant  Value=0.75
  Demux : Demux  Outputs=3
  Demux1 : Demux  Outputs=2
  Multiply : Product  Inputs=3
  Mux : Mux  Inputs=3
  Square : Math  Operator=square  SignedPower=on  SaturateOnIntegerOverflow=on
  Square1 : Math  Operator=square  SignedPower=on  SaturateOnIntegerOverflow=on
  Square2 : Math  Operator=square  SignedPower=on  SaturateOnIntegerOverflow=on
  Sum : Sum  Inputs=+++
  Terminator : Terminator
  Terminator1 : Terminator
  Zero : Constant  Value=0  OutDataTypeStr=Inherit: Inherit via back propagation
  Drag Forces in Body Axis : Outport  VectorParamsAs1DForOutWhenUnconnected=off
  wires:
  AOA and Side Slip/1 -> Demux1/1
  Marine Velocities in Body Axis/1 -> Demux/1
  Mux/1 -> Drag Forces in Body Axis/1
  Square2/1 -> Sum/3
  Demux/3 -> Square2/1  "Heave"
  Sum/1 -> Multiply/1
  Demux/1 -> Square/1  "Surge"
  Demux/2 -> Square1/1  "Sway"
  Square/1 -> Sum/2
  Square1/1 -> Sum/1
  Demux1/1 -> Terminator/1
  Demux1/2 -> Terminator1/1
  Constant/1 -> Multiply/2
  Constant1/1 -> Multiply/3
  Multiply/1 -> Mux/1
  Zero/1 -> Mux/3, Mux/2

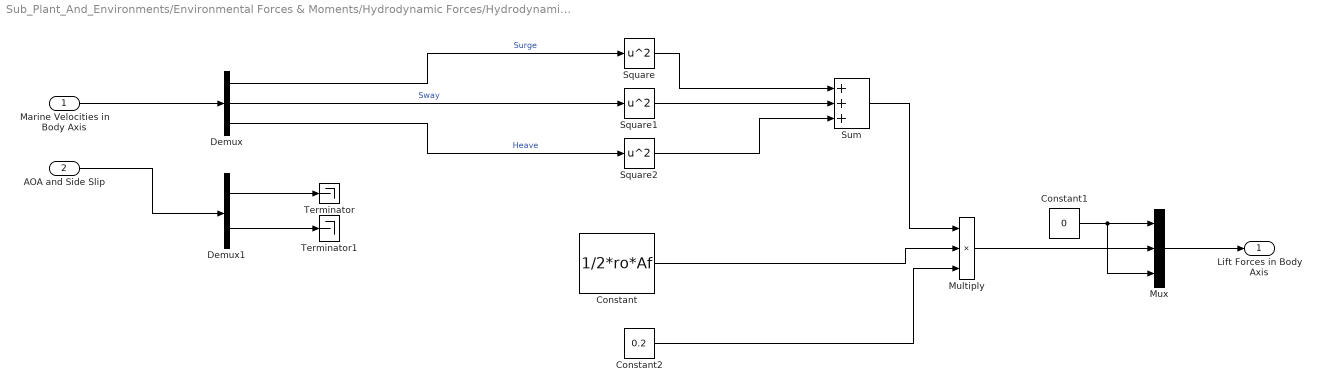
== system Sub_Plant_And_Environments/Environmental Forces & Moments/Hydrodynamic Forces/Hydrodynamic Forces - Basic/Force Exerted due to Lift (Body Axis) ==
  Marine Velocities in Body Axis : Inport
  AOA and Side Slip : Inport  Port=2
  Constant : Constant  Value=1/2*ro*Af  mask{ro=rho, Af=AF(1)}
      mask prompts: ro "Density of Water"; Af "Submarine Frontal Area"
      mask DialogControl DescGroupVar Prompt: Input
      mask DialogControl DescTextVar Prompt: Enter the following values :
  Constant1 : Constant  Value=0
  Constant2 : Constant  Value=0.2
  Demux : Demux  Outputs=3
  Demux1 : Demux  Outputs=2
  Multiply : Product  Inputs=3
  Mux : Mux  Inputs=3
  Square : Math  Operator=square  SignedPower=on  SaturateOnIntegerOverflow=on
  Square1 : Math  Operator=square  SignedPower=on  SaturateOnIntegerOverflow=on
  Square2 : Math  Operator=square  SignedPower=on  SaturateOnIntegerOverflow=on
  Sum : Sum  Inputs=+++
  Terminator : Terminator
  Terminator1 : Terminator
  Lift Forces in Body Axis : Outport  VectorParamsAs1DForOutWhenUnconnected=off
  wires:
  Constant1/1 -> Mux/3, Mux/1
  Square/1 -> Sum/1
  Demux/2 -> Square1/1  "Sway"
  Demux/1 -> Square/1  "Surge"
  Demux/3 -> Square2/1  "Heave"
  Square2/1 -> Sum/3
  Mux/1 -> Lift Forces in Body Axis/1
  Marine Velocities in Body Axis/1 -> Demux/1
  AOA and Side Slip/1 -> Demux1/1
  Square1/1 -> Sum/2
  Sum/1 -> Multiply/1
  Constant/1 -> Multiply/2
  Constant2/1 -> Multiply/3
  Multiply/1 -> Mux/2
  Demux1/1 -> Terminator/1
  Demux1/2 -> Terminator1/1

== system Sub_Plant_And_Environments/Environmental Forces & Moments/Hydrostatic Forces/Environment Model/3D Rotate Drag ==
  Force : Inport
  "Roll, Pitch, Yaw" : Inport  Port=2
  Gain : Gain
  Matrix Multiply : Product  Multiplication=Matrix(*)
  Rotation Angles to Direction Cosine Matrix : sharedtransform/Rotation Angles to Direction Cosine Matrix  rotationOrder=XYZ  aMode=aMode
      settings: SourceProductBaseCode=AE,PW,MT,VE,VP
  Transpose : Math  Operator=transpose  SignedPower=on  SaturateOnIntegerOverflow=on
  "Transformed_Force " : Outport  VectorParamsAs1DForOutWhenUnconnected=off
  wires:
  Matrix Multiply/1 -> "Transformed_Force "/1
  Rotation Angles to Direction Cosine Matrix/1 -> Transpose/1
  Force/1 -> Matrix Multiply/2
  "Roll, Pitch, Yaw"/1 -> Gain/1
  Transpose/1 -> Matrix Multiply/1
  Gain/1 -> Rotation Angles to Direction Cosine Matrix/1

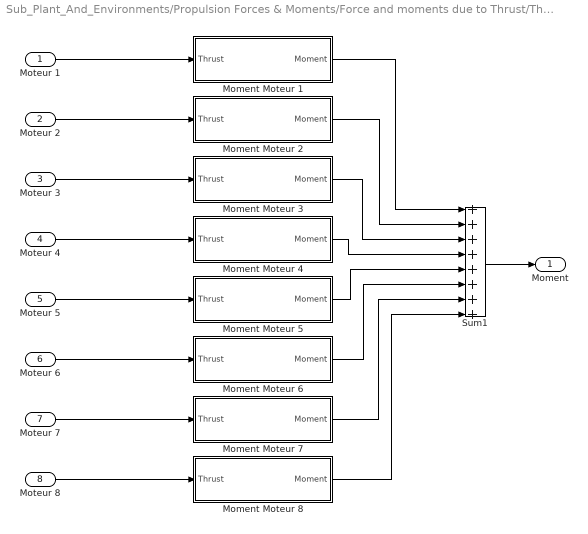
== system Sub_Plant_And_Environments/Propulsion Forces & Moments/Force and moments due to Thrust/Thrust to Propulsion /Moment computation ==
  Moteur 1 : Inport
  Moteur 2 : Inport  Port=2
  Moteur 3 : Inport  Port=3
  Moteur 4 : Inport  Port=4
  Moteur 5 : Inport  Port=5
  Moteur 6 : Inport  Port=6
  Moteur 7 : Inport  Port=7
  Moteur 8 : Inport  Port=8
  Moment Moteur 1 : Subsystem  mask{a=l1(1), b=l1(2), c=l1(3)}
      mask prompts: a "X Coordinate of Thruster from Center of Buoyancy"; b "Y Coordinate of Thruster from Center of Buoyancy"; c "Z Coordinate of Thruster from Center of Buoyancy"
      mask DialogControl DescTextVar Prompt: Enter Thruster Position w.r.t Center of Buoyancy
  Moment Moteur 2 : Subsystem  mask{a=l2(1), b=l2(2), c=l2(3)}
      mask prompts: a "X Coordinate of Thruster from Center of Buoyancy"; b "Y Coordinate of Thruster from Center of Buoyancy"; c "Z Coordinate of Thruster from Center of Buoyancy"
      mask DialogControl DescTextVar Prompt: Enter Thruster Position w.r.t Center of Buoyancy
  Moment Moteur 3 : Subsystem  mask{a=l3(1), b=l3(2), c=l3(3)}
      mask prompts: a "X Coordinate of Thruster from Center of Buoyancy"; b "Y Coordinate of Thruster from Center of Buoyancy"; c "Z Coordinate of Thruster from Center of Buoyancy"
      mask DialogControl DescTextVar Prompt: Enter Thruster Position w.r.t Center of Buoyancy
  Moment Moteur 4 : Subsystem  mask{a=l4(1), b=l4(2), c=l4(3)}
      mask prompts: a "X Coordinate of Thruster from Center of Buoyancy"; b "Y Coordinate of Thruster from Center of Buoyancy"; c "Z Coordinate of Thruster from Center of Buoyancy"
      mask DialogControl DescTextVar Prompt: Enter Thruster Position w.r.t Center of Buoyancy
  Moment Moteur 5 : Subsystem  mask{a=l5(1), b=l5(2), c=l5(3)}
      mask prompts: a "X Coordinate of Thruster from Center of Buoyancy"; b "Y Coordinate of Thruster from Center of Buoyancy"; c "Z Coordinate of Thruster from Center of Buoyancy"
      mask DialogControl DescTextVar Prompt: Enter Thruster Position w.r.t Center of Buoyancy
  Moment Moteur 6 : Subsystem  mask{a=l6(1), b=l6(2), c=l6(3)}
      mask prompts: a "X Coordinate of Thruster from Center of Buoyancy"; b "Y Coordinate of Thruster from Center of Buoyancy"; c "Z Coordinate of Thruster from Center of Buoyancy"
      mask DialogControl DescTextVar Prompt: Enter Thruster Position w.r.t Center of Buoyancy
  Moment Moteur 7 : Subsystem  mask{a=l7(1), b=l7(2), c=l7(3)}
      mask prompts: a "X Coordinate of Thruster from Center of Buoyancy"; b "Y Coordinate of Thruster from Center of Buoyancy"; c "Z Coordinate of Thruster from Center of Buoyancy"
      mask DialogControl DescTextVar Prompt: Enter Thruster Position w.r.t Center of Buoyancy
  Moment Moteur 8 : Subsystem  mask{a=l8(1), b=l8(2), c=l8(3)}
      mask prompts: a "X Coordinate of Thruster from Center of Buoyancy"; b "Y Coordinate of Thruster from Center of Buoyancy"; c "Z Coordinate of Thruster from Center of Buoyancy"
      mask DialogControl DescTextVar Prompt: Enter Thruster Position w.r.t Center of Buoyancy
  Sum1 : Sum  Inputs=++++++++
  Moment : Outport  VectorParamsAs1DForOutWhenUnconnected=off
  wires:
  Moteur 4/1 -> Moment Moteur 4/1(Thrust)
  Moteur 1/1 -> Moment Moteur 1/1(Thrust)
  Moteur 3/1 -> Moment Moteur 3/1(Thrust)
  Moment Moteur 1/1(Moment) -> Sum1/1
  Moment Moteur 2/1(Moment) -> Sum1/2
  Moment Moteur 5/1(Moment) -> Sum1/5
  Moment Moteur 4/1(Moment) -> Sum1/4
  Moteur 5/1 -> Moment Moteur 5/1(Thrust)
  Moment Moteur 3/1(Moment) -> Sum1/3
  Sum1/1 -> Moment/1
  Moteur 2/1 -> Moment Moteur 2/1(Thrust)
  Moment Moteur 6/1(Moment) -> Sum1/6
  Moteur 6/1 -> Moment Moteur 6/1(Thrust)
  Moment Moteur 7/1(Moment) -> Sum1/7
  Moteur 7/1 -> Moment Moteur 7/1(Thrust)
  Moment Moteur 8/1(Moment) -> Sum1/8
  Moteur 8/1 -> Moment Moteur 8/1(Thrust)

== system Sub_Plant_And_Environments/Propulsion Forces & Moments/Force and moments due to Thrust/Thrust to Propulsion /Thrust Transformation ==
  Thrust Inputs : Inport
  Demux1 : Demux  Outputs=8
  Thrust M1 : Outport  VectorParamsAs1DForOutWhenUnconnected=off
  Thrust M2 : Outport  Port=2  VectorParamsAs1DForOutWhenUnconnected=off
  Thrust M3 : Outport  Port=3  VectorParamsAs1DForOutWhenUnconnected=off
  Thrust M4 : Outport  Port=4  VectorParamsAs1DForOutWhenUnconnected=off
  Thrust M5 : Outport  Port=5  VectorParamsAs1DForOutWhenUnconnected=off
  Thrust M6 : Outport  Port=6  VectorParamsAs1DForOutWhenUnconnected=off
  Thrust M7 : Outport  Port=7  VectorParamsAs1DForOutWhenUnconnected=off
  Thrust M8 : Outport  Port=8  VectorParamsAs1DForOutWhenUnconnected=off
  wires:
  Demux1/4 -> Thrust M4/1
  Demux1/5 -> Thrust M5/1
  Thrust Inputs/1 -> Demux1/1
  Demux1/1 -> Thrust M1/1
  Demux1/2 -> Thrust M2/1
  Demux1/3 -> Thrust M3/1
  Demux1/6 -> Thrust M6/1
  Demux1/7 -> Thrust M7/1
  Demux1/8 -> Thrust M8/1

== system Sub_Plant_And_Environments/Propulsion Forces & Moments/Input commands to Thrust/PWM Signals to Thrust /Thrust_direction Moteur 1 ==
  Thrust : Inport
  Constant3 : Constant  Value=a_rad(1,:)
  Matrix Multiply : Product  Multiplication=Matrix(*)
  Rotation Angles to Direction Cosine Matrix : sharedtransform/Rotation Angles to Direction Cosine Matrix  rotationOrder=ZYX  aMode=aMode
      settings: SourceProductBaseCode=AE,PW,MT,VE,VP
  Transpose : Math  Operator=transpose  SignedPower=on  SaturateOnIntegerOverflow=on
  "Transformed_Thrust " : Outport  VectorParamsAs1DForOutWhenUnconnected=off
  wires:
  Matrix Multiply/1 -> "Transformed_Thrust "/1
  Rotation Angles to Direction Cosine Matrix/1 -> Transpose/1
  Thrust/1 -> Matrix Multiply/2
  Transpose/1 -> Matrix Multiply/1
  Constant3/1 -> Rotation Angles to Direction Cosine Matrix/1

== system Sub_Plant_And_Environments/Propulsion Forces & Moments/Input commands to Thrust/PWM Signals to Thrust /Thrust_direction Moteur 2 ==
  Thrust : Inport
  Constant : Constant  Value=a_rad(2,:)
  Matrix Multiply : Product  Multiplication=Matrix(*)
  Rotation Angles to Direction Cosine Matrix : sharedtransform/Rotation Angles to Direction Cosine Matrix  rotationOrder=ZYX  aMode=aMode
      settings: SourceProductBaseCode=AE,PW,MT,VE,VP
  Transpose : Math  Operator=transpose  SignedPower=on  SaturateOnIntegerOverflow=on
  "Transformed_Thrust " : Outport  VectorParamsAs1DForOutWhenUnconnected=off
  wires:
  Matrix Multiply/1 -> "Transformed_Thrust "/1
  Rotation Angles to Direction Cosine Matrix/1 -> Transpose/1
  Thrust/1 -> Matrix Multiply/2
  Transpose/1 -> Matrix Multiply/1
  Constant/1 -> Rotation Angles to Direction Cosine Matrix/1

== system Sub_Plant_And_Environments/Propulsion Forces & Moments/Input commands to Thrust/PWM Signals to Thrust /Thrust_direction Moteur 3 ==
  Thrust : Inport
  Constant : Constant  Value=a_rad(3,:)
  Matrix Multiply : Product  Multiplication=Matrix(*)
  Rotation Angles to Direction Cosine Matrix : sharedtransform/Rotation Angles to Direction Cosine Matrix  rotationOrder=ZYX  aMode=aMode
      settings: SourceProductBaseCode=AE,PW,MT,VE,VP
  Transpose : Math  Operator=transpose  SignedPower=on  SaturateOnIntegerOverflow=on
  "Transformed_Thrust " : Outport  VectorParamsAs1DForOutWhenUnconnected=off
  wires:
  Matrix Multiply/1 -> "Transformed_Thrust "/1
  Rotation Angles to Direction Cosine Matrix/1 -> Transpose/1
  Thrust/1 -> Matrix Multiply/2
  Transpose/1 -> Matrix Multiply/1
  Constant/1 -> Rotation Angles to Direction Cosine Matrix/1

== system Sub_Plant_And_Environments/Propulsion Forces & Moments/Input commands to Thrust/PWM Signals to Thrust /Thrust_direction Moteur 4 ==
  Thrust : Inport
  Constant : Constant  Value=a_rad(4,:)
  Matrix Multiply : Product  Multiplication=Matrix(*)
  Rotation Angles to Direction Cosine Matrix : sharedtransform/Rotation Angles to Direction Cosine Matrix  rotationOrder=ZYX  aMode=aMode
      settings: SourceProductBaseCode=AE,PW,MT,VE,VP
  Transpose : Math  Operator=transpose  SignedPower=on  SaturateOnIntegerOverflow=on
  "Transformed_Thrust " : Outport  VectorParamsAs1DForOutWhenUnconnected=off
  wires:
  Matrix Multiply/1 -> "Transformed_Thrust "/1
  Rotation Angles to Direction Cosine Matrix/1 -> Transpose/1
  Thrust/1 -> Matrix Multiply/2
  Transpose/1 -> Matrix Multiply/1
  Constant/1 -> Rotation Angles to Direction Cosine Matrix/1

== system Sub_Plant_And_Environments/Propulsion Forces & Moments/Input commands to Thrust/PWM Signals to Thrust /Thrust_direction Moteur 5 ==
  Thrust : Inport
  Constant : Constant  Value=a_rad(5,:)
  Matrix Multiply : Product  Multiplication=Matrix(*)
  Rotation Angles to Direction Cosine Matrix : sharedtransform/Rotation Angles to Direction Cosine Matrix  rotationOrder=ZYX  aMode=aMode
      settings: SourceProductBaseCode=AE,PW,MT,VE,VP
  Transpose : Math  Operator=transpose  SignedPower=on  SaturateOnIntegerOverflow=on
  "Transformed_Thrust " : Outport  VectorParamsAs1DForOutWhenUnconnected=off
  wires:
  Matrix Multiply/1 -> "Transformed_Thrust "/1
  Rotation Angles to Direction Cosine Matrix/1 -> Transpose/1
  Thrust/1 -> Matrix Multiply/2
  Transpose/1 -> Matrix Multiply/1
  Constant/1 -> Rotation Angles to Direction Cosine Matrix/1

== system Sub_Plant_And_Environments/Propulsion Forces & Moments/Input commands to Thrust/PWM Signals to Thrust /Thrust_direction Moteur 6 ==
  Thrust : Inport
  Constant : Constant  Value=a_rad(6,:)
  Matrix Multiply : Product  Multiplication=Matrix(*)
  Rotation Angles to Direction Cosine Matrix : sharedtransform/Rotation Angles to Direction Cosine Matrix  rotationOrder=ZYX  aMode=aMode
      settings: SourceProductBaseCode=AE,PW,MT,VE,VP
  Transpose : Math  Operator=transpose  SignedPower=on  SaturateOnIntegerOverflow=on
  "Transformed_Thrust " : Outport  VectorParamsAs1DForOutWhenUnconnected=off
  wires:
  Matrix Multiply/1 -> "Transformed_Thrust "/1
  Rotation Angles to Direction Cosine Matrix/1 -> Transpose/1
  Thrust/1 -> Matrix Multiply/2
  Transpose/1 -> Matrix Multiply/1
  Constant/1 -> Rotation Angles to Direction Cosine Matrix/1

== system Sub_Plant_And_Environments/Propulsion Forces & Moments/Input commands to Thrust/PWM Signals to Thrust /Thrust_direction Moteur 7 ==
  Thrust : Inport
  Constant : Constant  Value=a_rad(7,:)
  Matrix Multiply : Product  Multiplication=Matrix(*)
  Rotation Angles to Direction Cosine Matrix : sharedtransform/Rotation Angles to Direction Cosine Matrix  rotationOrder=ZYX  aMode=aMode
      settings: SourceProductBaseCode=AE,PW,MT,VE,VP
  Transpose : Math  Operator=transpose  SignedPower=on  SaturateOnIntegerOverflow=on
  "Transformed_Thrust " : Outport  VectorParamsAs1DForOutWhenUnconnected=off
  wires:
  Matrix Multiply/1 -> "Transformed_Thrust "/1
  Rotation Angles to Direction Cosine Matrix/1 -> Transpose/1
  Thrust/1 -> Matrix Multiply/2
  Transpose/1 -> Matrix Multiply/1
  Constant/1 -> Rotation Angles to Direction Cosine Matrix/1

== system Sub_Plant_And_Environments/Propulsion Forces & Moments/Input commands to Thrust/PWM Signals to Thrust /Thrust_direction Moteur 8 ==
  Thrust : Inport
  Constant : Constant  Value=a_rad(8,:)
  Matrix Multiply : Product  Multiplication=Matrix(*)
  Rotation Angles to Direction Cosine Matrix : sharedtransform/Rotation Angles to Direction Cosine Matrix  rotationOrder=ZYX  aMode=aMode
      settings: SourceProductBaseCode=AE,PW,MT,VE,VP
  Transpose : Math  Operator=transpose  SignedPower=on  SaturateOnIntegerOverflow=on
  "Transformed_Thrust " : Outport  VectorParamsAs1DForOutWhenUnconnected=off
  wires:
  Matrix Multiply/1 -> "Transformed_Thrust "/1
  Rotation Angles to Direction Cosine Matrix/1 -> Transpose/1
  Thrust/1 -> Matrix Multiply/2
  Transpose/1 -> Matrix Multiply/1
  Constant/1 -> Rotation Angles to Direction Cosine Matrix/1

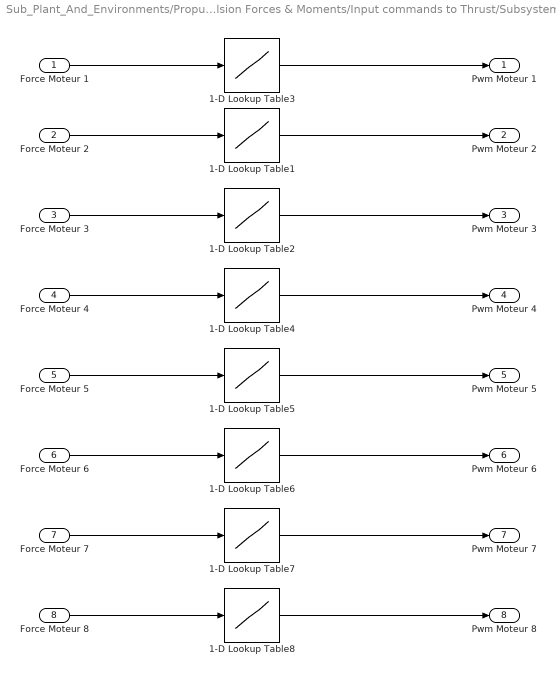
== system Sub_Plant_And_Environments/Propulsion Forces & Moments/Input commands to Thrust/Subsystem/Input Forces to PWM ==
  Force Moteur 1 : Inport
  Force Moteur 2 : Inport  Port=2
  Force Moteur 3 : Inport  Port=3
  Force Moteur 4 : Inport  Port=4
  Force Moteur 5 : Inport  Port=5
  Force Moteur 6 : Inport  Port=6
  Force Moteur 7 : Inport  Port=7
  Force Moteur 8 : Inport  Port=8
  1-D Lookup Table{1..8} (8 alike) : Lookup_n-D  NumberOfTableDimensions=1  BreakpointsForDimension1=N  Table=PWM  InternalRulePriority=Speed  RndMeth=Simplest  InputSameDT=on
  Pwm Moteur 1 : Outport  VectorParamsAs1DForOutWhenUnconnected=off
  Pwm Moteur 2 : Outport  Port=2  VectorParamsAs1DForOutWhenUnconnected=off
  Pwm Moteur 3 : Outport  Port=3  VectorParamsAs1DForOutWhenUnconnected=off
  Pwm Moteur 4 : Outport  Port=4  VectorParamsAs1DForOutWhenUnconnected=off
  Pwm Moteur 5 : Outport  Port=5  VectorParamsAs1DForOutWhenUnconnected=off
  Pwm Moteur 6 : Outport  Port=6  VectorParamsAs1DForOutWhenUnconnected=off
  Pwm Moteur 7 : Outport  Port=7  VectorParamsAs1DForOutWhenUnconnected=off
  Pwm Moteur 8 : Outport  Port=8  VectorParamsAs1DForOutWhenUnconnected=off
  wires:
  1-D Lookup Table3/1 -> Pwm Moteur 1/1
  Force Moteur 1/1 -> 1-D Lookup Table3/1
  1-D Lookup Table1/1 -> Pwm Moteur 2/1
  Force Moteur 2/1 -> 1-D Lookup Table1/1
  1-D Lookup Table2/1 -> Pwm Moteur 3/1
  Force Moteur 3/1 -> 1-D Lookup Table2/1
  1-D Lookup Table4/1 -> Pwm Moteur 4/1
  Force Moteur 4/1 -> 1-D Lookup Table4/1
  1-D Lookup Table5/1 -> Pwm Moteur 5/1
  Force Moteur 5/1 -> 1-D Lookup Table5/1
  1-D Lookup Table6/1 -> Pwm Moteur 6/1
  Force Moteur 6/1 -> 1-D Lookup Table6/1
  1-D Lookup Table7/1 -> Pwm Moteur 7/1
  Force Moteur 7/1 -> 1-D Lookup Table7/1
  1-D Lookup Table8/1 -> Pwm Moteur 8/1
  Force Moteur 8/1 -> 1-D Lookup Table8/1

== system Sub_Plant_And_Environments/Propulsion Forces & Moments/Force and moments due to Thrust/Thrust to Propulsion /Moment computation/Moment Moteur 1 ==
  Thrust : Inport
  Constant : Constant  Value=[a;b;c]
  Cross Product : vrlib/Utilities/Cross Product
  Moment : Outport  VectorParamsAs1DForOutWhenUnconnected=off
  wires:
  Cross Product/1 -> Moment/1
  Thrust/1 -> Cross Product/2
  Constant/1 -> Cross Product/1

== system Sub_Plant_And_Environments/Propulsion Forces & Moments/Force and moments due to Thrust/Thrust to Propulsion /Moment computation/Moment Moteur 2 ==
  Thrust : Inport
  Constant : Constant  Value=[a;b;c]
  Cross Product : vrlib/Utilities/Cross Product
  Moment : Outport  VectorParamsAs1DForOutWhenUnconnected=off
  wires:
  Constant/1 -> Cross Product/1
  Thrust/1 -> Cross Product/2
  Cross Product/1 -> Moment/1

== system Sub_Plant_And_Environments/Propulsion Forces & Moments/Force and moments due to Thrust/Thrust to Propulsion /Moment computation/Moment Moteur 3 ==
  Thrust : Inport
  Constant : Constant  Value=[a;b;c]
  Cross Product : vrlib/Utilities/Cross Product
  Moment : Outport  VectorParamsAs1DForOutWhenUnconnected=off
  wires:
  Cross Product/1 -> Moment/1
  Thrust/1 -> Cross Product/2
  Constant/1 -> Cross Product/1

== system Sub_Plant_And_Environments/Propulsion Forces & Moments/Force and moments due to Thrust/Thrust to Propulsion /Moment computation/Moment Moteur 4 ==
  Thrust : Inport
  Constant : Constant  Value=[a;b;c]
  Cross Product : vrlib/Utilities/Cross Product
  Moment : Outport  VectorParamsAs1DForOutWhenUnconnected=off
  wires:
  Constant/1 -> Cross Product/1
  Thrust/1 -> Cross Product/2
  Cross Product/1 -> Moment/1

== system Sub_Plant_And_Environments/Propulsion Forces & Moments/Force and moments due to Thrust/Thrust to Propulsion /Moment computation/Moment Moteur 5 ==
  Thrust : Inport
  Constant : Constant  Value=[a;b;c]
  Cross Product : vrlib/Utilities/Cross Product
  Moment : Outport  VectorParamsAs1DForOutWhenUnconnected=off
  wires:
  Cross Product/1 -> Moment/1
  Thrust/1 -> Cross Product/2
  Constant/1 -> Cross Product/1

== system Sub_Plant_And_Environments/Propulsion Forces & Moments/Force and moments due to Thrust/Thrust to Propulsion /Moment computation/Moment Moteur 6 ==
  Thrust : Inport
  Constant : Constant  Value=[a;b;c]
  Cross Product : vrlib/Utilities/Cross Product
  Moment : Outport  VectorParamsAs1DForOutWhenUnconnected=off
  wires:
  Cross Product/1 -> Moment/1
  Thrust/1 -> Cross Product/2
  Constant/1 -> Cross Product/1

== system Sub_Plant_And_Environments/Propulsion Forces & Moments/Force and moments due to Thrust/Thrust to Propulsion /Moment computation/Moment Moteur 7 ==
  Thrust : Inport
  Constant : Constant  Value=[a;b;c]
  Cross Product : vrlib/Utilities/Cross Product
  Moment : Outport  VectorParamsAs1DForOutWhenUnconnected=off
  wires:
  Cross Product/1 -> Moment/1
  Thrust/1 -> Cross Product/2
  Constant/1 -> Cross Product/1
